simulink subsystem "Kinematics"  (R2021a)
settings: Solver=VariableStepAuto  StartTime=0.0  StopTime=10.0  RelTol=1e-3
undefined symbols (not defined in the file): n, q0, r0
libraries: aerolibutil x3
settings Model: Creator=Laura  LastModifiedBy=Laura

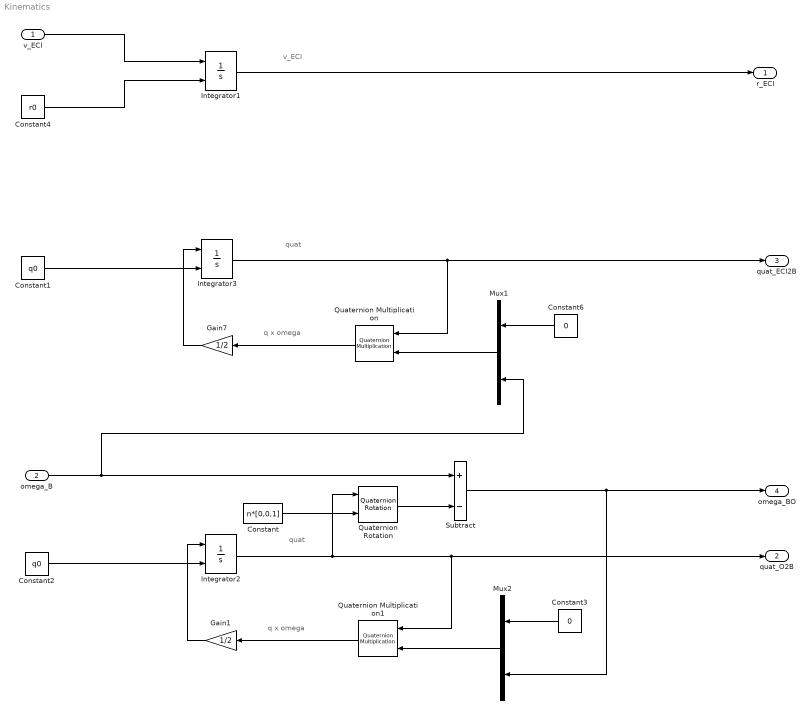
== system Kinematics ==
  note: v_ECI
  note: quat
  note: q x omega
  note: quat
  note: q x omega
  v_ECI : Inport
  omega_B : Inport  Port=2
  Constant : Constant  Value=n*[0,0,1]
  Constant1 : Constant  Value=q0
  Constant2 : Constant  Value=q0
  Constant3 : Constant  Value=0
  Constant4 : Constant  Value=r0
  Constant6 : Constant  Value=0
  Gain1 : Gain  Gain=1/2
  Gain7 : Gain  Gain=1/2
  Integrator1 : Integrator  InitialConditionSource=external
  Integrator2 : Integrator  InitialConditionSource=external
  Integrator3 : Integrator  InitialConditionSource=external
  Mux1 : Mux  Inputs=2
  Mux2 : Mux  Inputs=2
  Quaternion Multiplication : aerolibutil/Quaternion Multiplication
  Quaternion Multiplication1 : aerolibutil/Quaternion Multiplication
  Quaternion Rotation : aerolibutil/Quaternion Rotation
  Subtract : Sum  Inputs=+-
  r_ECI : Outport
  quat_O2B : Outport  Port=2
  quat_ECI2B : Outport  Port=3
  omega_BO : Outport  Port=4
  wires:
  Integrator3/1 -> Quaternion Multiplication/1, quat_ECI2B/1
  Mux1/1 -> Quaternion Multiplication/2
  Integrator1/1 -> r_ECI/1
  Gain7/1 -> Integrator3/1
  Constant4/1 -> Integrator1/2
  Constant6/1 -> Mux1/1
  Constant1/1 -> Integrator3/2
  Quaternion Multiplication/1 -> Gain7/1
  v_ECI/1 -> Integrator1/1
  Mux2/1 -> Quaternion Multiplication1/2
  Gain1/1 -> Integrator2/1
  Constant3/1 -> Mux2/1
  Quaternion Multiplication1/1 -> Gain1/1
  Constant2/1 -> Integrator2/2
  omega_B/1 -> Mux1/2, Subtract/1
  Quaternion Rotation/1 -> Subtract/2
  Constant/1 -> Quaternion Rotation/2
  Subtract/1 -> omega_BO/1, Mux2/2
  Integrator2/1 -> Quaternion Multiplication1/1, quat_O2B/1, Quaternion Rotation/1
